simulink model "Rotor_position"  (R2020a)
settings: Solver=ode4  StartTime=0.0  StopTime=2  FixedStep=1e-4  RelTol=1e-3
settings Model: Creator=samee
settings DebuggingCC: UnconnectedInputMsg=none  UnconnectedOutputMsg=none  UnconnectedLineMsg=none

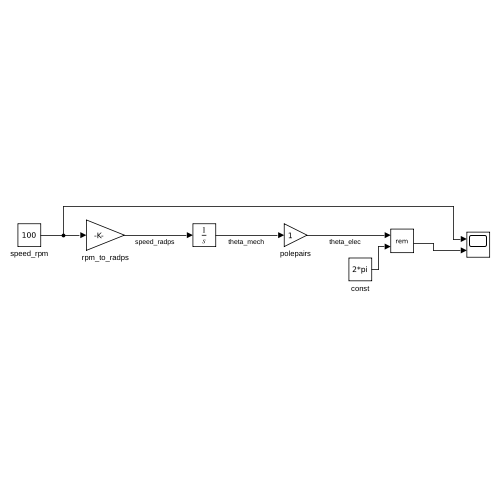
[thumbnail: Simulink's stored preview of the top-level diagram]
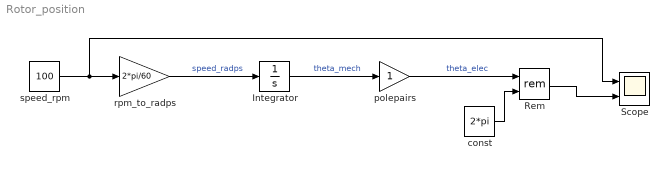
== system Rotor_position ==
  Integrator : Integrator
  Rem : Math  Operator=rem  SaturateOnIntegerOverflow=on
  Scope : Scope  NumInputPorts=2
  const : Constant  Value=2*pi
  polepairs : Gain
  rpm_to_radps : Gain  Gain=2*pi/60
  speed_rpm : Constant  Value=100
  wires:
  speed_rpm/1 -> Scope/1, rpm_to_radps/1
  Integrator/1 -> polepairs/1  "theta_mech"
  rpm_to_radps/1 -> Integrator/1  "speed_radps"
  polepairs/1 -> Rem/1  "theta_elec"
  const/1 -> Rem/2
  Rem/1 -> Scope/2
